simulink model "PV_Array_With_Faults"  (R2023b)
settings: Solver=FixedStepAuto  StartTime=1  StopTime=1440  FixedStep=1  RelTol=1e-3
libraries: spsSeriesRLCBranchLib x5, spsIdealSwitchLib x3, spsCurrentMeasurementLib x1, spsDiodeLib x1, spsMosfetLib x1, spsPVArrayLib x1, eePwmGenerator x1, spsVoltageMeasurementLib x1, spspowerguiLib x1
settings Model: NumberOfSteps=10  Creator=chate  LastModifiedBy=chate

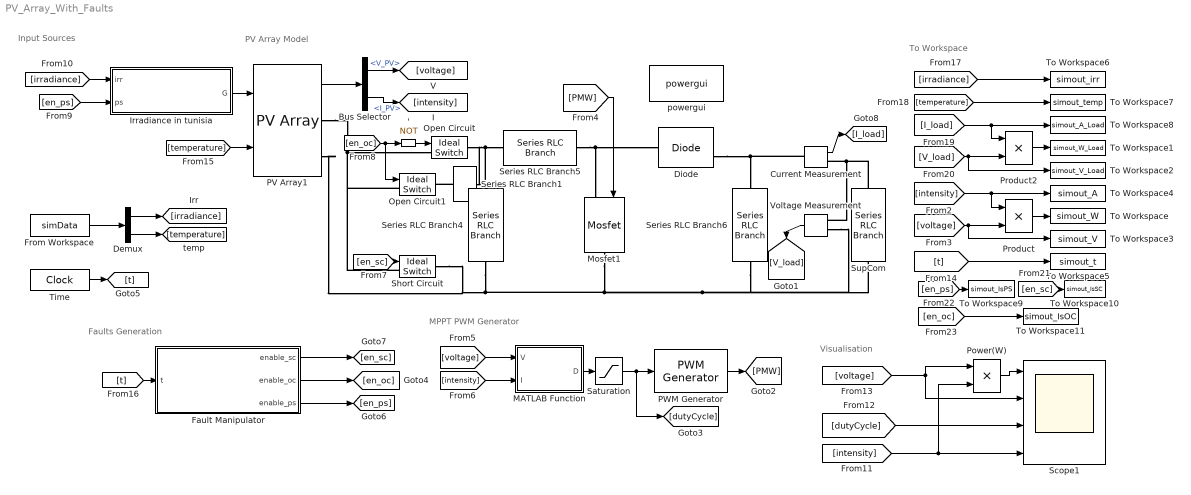
== system PV_Array_With_Faults ==
  note: Input Sources
  note: PV Array Model
  note: Faults Generation
  note: To Workspace
  note: MPPT PWM Generator
  note: Visualisation
  ' : Logic  Operator=NOT  IconShape=distinctive  AllPortsSameDT=off  OutDataTypeStr=boolean
  Bus Selector : BusSelector  OutputSignals=V_PV,I_PV
  Current Measurement : spsCurrentMeasurementLib/Current Measurement  PhasorSimulation=off  OutputType=Complex  PSBequivalent=0
  Demux : Demux  Outputs=2
  Diode : spsDiodeLib/Diode  Ron=0.001  Lon=0  Vf=0.8  IC=0  UseSnubber=0  Rs=100  Cs=1e-7  Measurements=on
  Fault Manipulator : MATLAB Function  TreatAsAtomicUnit=on
  From Workspace : FromWorkspace  VariableName=simData  OutputAfterFinalValue=Setting to zero
  Irradiance in tunisia : MATLAB Function  TreatAsAtomicUnit=on
  MATLAB Function : MATLAB Function  TreatAsAtomicUnit=on
  Mosfet1 : spsMosfetLib/Mosfet  Ron=1e-3  Lon=0  Rd=1e-3  Vfd=0  IC=0  Rs=100  Cs=1e-7  Measurements=off
  Open Circuit : spsIdealSwitchLib/Ideal Switch  Ron=0.000001  Lon=0  IC=1  Rs=0  Cs=0  Measurements=off
  Open Circuit1 : spsIdealSwitchLib/Ideal Switch  Ron=0.000001  Lon=0  IC=0  Rs=0  Cs=0  Measurements=off
  PV Array1 : spsPVArrayLib/PV Array  Npar=3  Nser=15  PlotType=array @ 1000 W/m2 & specified temperatures  S_vec="[ 1000  500  100 ]"  Temp_C_vec="[ 45 25  ]"  ModuleName=User-defined  PlotWhenSelected=off  Pm=451.278  Ncell=60  Voc=49.8  Isc=11.56  Vm=41.1  Im=10.98  beta_Voc_pc=-0.36099  alpha_Isc_pc=0.102  beta_Voc=-0.17977  alpha_Isc=0.011791  IL=11.6189  I0=4.2897e-10  nI=1.3452  Rsh=602.3017  Rs=0.22981  RobustModel=off  RobustCellTemperature=25  BAL=on  Tc=1e-6  Tfilter=5e-5
  PWM Generator : eePwmGenerator/PWM Generator  CarrCount=Up  Tper=864000  Tdelay=0  Ts=86400
  Power(W) : Product
  Product : Product
  Product2 : Product
  Saturation : Saturate  UpperLimit=1  LowerLimit=0
  Scope1 : Scope  NumInputPorts=4
  Series RLC Branch1 : spsSeriesRLCBranchLib/Series RLC Branch  LConnTagsString=__new0  RConnTagsString=__new0  BranchType=R  Resistance=7.3  Inductance=1.63e-2  SetiL0=off  InitialCurrent=0  Capacitance=1e-3  Setx0=off  InitialVoltage=0  Measurements=None
  Series RLC Branch4 : spsSeriesRLCBranchLib/Series RLC Branch  LConnTagsString=__new0  RConnTagsString=__new0  BranchType=C  Resistance=1  Inductance=1e-3  SetiL0=off  InitialCurrent=0  Capacitance=46.6e-2  Setx0=off  InitialVoltage=0  Measurements=None
  Series RLC Branch5 : spsSeriesRLCBranchLib/Series RLC Branch  LConnTagsString=__new0  RConnTagsString=__new0  BranchType=L  Resistance=1  Inductance=1.63e-2  SetiL0=off  InitialCurrent=0  Capacitance=1e-3  Setx0=off  InitialVoltage=0  Measurements=None
  Series RLC Branch6 : spsSeriesRLCBranchLib/Series RLC Branch  LConnTagsString=__new0  RConnTagsString=__new0  BranchType=C  Resistance=1  Inductance=1e-3  SetiL0=off  InitialCurrent=0  Capacitance=63e-2  Setx0=off  InitialVoltage=0  Measurements=None
  Short Circuit : spsIdealSwitchLib/Ideal Switch  Ron=0.000001  Lon=0  IC=0  Rs=0  Cs=0  Measurements=off
  SupCom : spsSeriesRLCBranchLib/Series RLC Branch  LConnTagsString=__new0  RConnTagsString=__new0  BranchType=R  Resistance=18.5  Inductance=1e-3  SetiL0=off  InitialCurrent=0  Capacitance=1e-3  Setx0=off  InitialVoltage=0  Measurements=None
  Time : DigitalClock
  To Workspace : ToWorkspace  VariableName=simout_W  SaveFormat=Timeseries  SampleTime=-1
  To Workspace1 : ToWorkspace  VariableName=simout_W_Load  SaveFormat=Timeseries  SampleTime=-1
  To Workspace10 : ToWorkspace  VariableName=simout_IsSC  SaveFormat=Timeseries  SampleTime=-1
  To Workspace11 : ToWorkspace  VariableName=simout_IsOC  SaveFormat=Timeseries  SampleTime=-1
  To Workspace2 : ToWorkspace  VariableName=simout_V_Load  SaveFormat=Timeseries  SampleTime=-1
  To Workspace3 : ToWorkspace  VariableName=simout_V  SaveFormat=Timeseries  SampleTime=-1
  To Workspace4 : ToWorkspace  VariableName=simout_A  SaveFormat=Timeseries  SampleTime=-1
  To Workspace5 : ToWorkspace  VariableName=simout_t  SaveFormat=Timeseries  SampleTime=-1
  To Workspace6 : ToWorkspace  VariableName=simout_irr  SaveFormat=Timeseries  SampleTime=-1
  To Workspace7 : ToWorkspace  VariableName=simout_temp  SaveFormat=Timeseries  SampleTime=-1
  To Workspace8 : ToWorkspace  VariableName=simout_A_Load  SaveFormat=Timeseries  SampleTime=-1
  To Workspace9 : ToWorkspace  VariableName=simout_IsPS  SaveFormat=Timeseries  SampleTime=-1
  Voltage Measurement : spsVoltageMeasurementLib/Voltage Measurement  PhasorSimulation=off  OutputType=Complex  PSBequivalent=0
  powergui : spspowerguiLib/powergui  Priority=1  SimulationMode=Discrete  SampleTime=1  frequency=60  Iterations=50  frequencyindice=0  Pbase=100e6  ErrMax=1e-4  UnitsV=kV  UnitsW=MW  buscounter=0  FunctionMessages=off  echomessages=off  EnableUseOfTLC=off  CurrentSourceSwitches=off  DisableSnubberDevices=off  DisableRonSwitches=off  DisableVfSwitches=off  DisplayEquations=off  AutomaticDiscreteSolvers=off  SolverType=Tustin/Backward Euler (TBE)  Interpol=off  ExternalGateDelay=off  methode=off  Ts=100  x0status=blocks  SPID=on  SwTol=0  HookPort=off  NonlinearTolerance=1e-4  nMaxIteration=100  ContinueOnMaxIteration=off  RestoreLinks=warning  ResistiveCurrentMeasurement=off  Frange=[0:2:500]  Ylog=off  Xlog=on  ShowGrid=off  save=off  variable=ZData  structure=0  ZoomFFT=off  StartTime=0.0  cycles=1  DisplayStyle=1  fundamental=60  FreqAxis=off  MaxFrequency=1000  frequencyindicesteady=1  RmsSteady=1  display=off
  wires:
  PV Array1/1 -> Bus Selector/1
  [intensity] -> Product/1, To Workspace4/1
  [voltage] -> To Workspace3/1, Product/2
  Product/1 -> To Workspace/1
  Bus Selector/1 -> [voltage]  "<V_PV>"
  Bus Selector/2 -> [intensity]  "<I_PV>"
  Voltage Measurement/1 -> [V_load]
  [PMW] -> Mosfet1/1
  MATLAB Function/1(D) -> Saturation/1
  PWM Generator/1 -> [PMW]
  [voltage] -> MATLAB Function/1(V)
  [intensity] -> MATLAB Function/2(I)
  [dutyCycle] -> Scope1/3
  [voltage] -> Power(W)/1, Scope1/2
  Power(W)/1 -> Scope1/1
  [intensity] -> Power(W)/2, Scope1/4
  Saturation/1 -> PWM Generator/1, [dutyCycle]
  Irradiance in tunisia/1(G) -> PV Array1/1
  [en_sc] -> Short Circuit/1
  Fault Manipulator/2(enable_oc) -> [en_oc]
  Fault Manipulator/1(enable_sc) -> [en_sc]
  [en_ps] -> Irradiance in tunisia/2(ps)
  Fault Manipulator/3(enable_ps) -> [en_ps]
  Time/1 -> [t]
  [t] -> To Workspace5/1
  [t] -> Fault Manipulator/1(t)
  Current Measurement/1 -> [I_load]
  [irradiance] -> To Workspace6/1
  [temperature] -> To Workspace7/1
  [V_load] -> To Workspace2/1, Product2/2
  Product2/1 -> To Workspace1/1
  [I_load] -> Product2/1, To Workspace8/1
  [en_ps] -> To Workspace9/1
  [en_sc] -> To Workspace10/1
  [en_oc] -> To Workspace11/1
  From Workspace/1 -> Demux/1
  Demux/2 -> [temperature]
  [temperature] -> PV Array1/2
  Demux/1 -> [irradiance]
  [irradiance] -> Irradiance in tunisia/1(irr)
  [en_oc] -> '/1, Open Circuit1/1
  '/1 -> Open Circuit/1
  connections:
  SupCom/LConn1 -- Current Measurement/RConn1 -- Voltage Measurement/LConn1
  Series RLC Branch4/RConn1 -- Short Circuit/RConn1 -- PV Array1/RConn2 -- Series RLC Branch6/RConn1 -- Voltage Measurement/LConn2 -- SupCom/RConn1 -- Mosfet1/RConn1
  Series RLC Branch5/RConn1 -- Mosfet1/LConn1 -- Diode/LConn1
  Current Measurement/LConn1 -- Diode/RConn1 -- Series RLC Branch6/LConn1
  Series RLC Branch4/LConn1 -- Series RLC Branch1/RConn1 -- Open Circuit/RConn1 -- Series RLC Branch5/LConn1
  PV Array1/RConn1 -- Open Circuit1/LConn1 -- Short Circuit/LConn1 -- Open Circuit/LConn1
  Series RLC Branch1/LConn1 -- Open Circuit1/RConn1

== matlab function PV_Array_With_Faults/Irradiance in tunisia ==
  data: irr input; G output; ps input
function G = irradiance_in_tunisia(irr, ps)
    
    G = max(0, irr);

    if ps == 1
        G = 0.85 * G;  % Reduce irradiance to 85%
    end
end

== matlab function PV_Array_With_Faults/Fault Manipulator ==
  data: t input; enable_sc output; enable_oc output; enable_ps output
function [enable_sc, enable_oc, enable_ps] = faults(t)
    % Time-dependent fault trigger system
    % Fault probability per second
    persistent fault_type fault_start_time fault_duration

    % Parameters
    fault_probability = 0.05;  % chance of a fault occurring at each call
    enable_sc = 0;
    enable_oc = 0;
    enable_ps = 0;

    % First call init
    if isempty(fault_type)
        fault_type = 0;
        fault_duration = 0;
        fault_start_time = -Inf;
    end

    % Check if current fault is active
    if t < fault_start_time + fault_duration
        % Maintain the current fault
        switch fault_type
            case 1
                enable_sc = 1;
                enable_oc = 0;
                enable_ps = 0;
            case 2
                enable_sc = 0;
                enable_oc = 1;
                enable_ps = 0;
            case 3
                enable_sc = 0;
                enable_oc = 0;
                enable_ps = 1;
        end
    else
        % No active fault, decide if a new one should start
        if rand < fault_probability
            fault_duration = randi(50) + 10;
            fault_type = randi(3);  % random fault (1=SC, 2=OC, 3=PS)
            fault_start_time = t;
        else
            % No fault
            fault_type = 0;
            enable_sc = 0;
            enable_oc = 0;
            enable_ps = 0;
        end
    end
end

== matlab function PV_Array_With_Faults/MATLAB Function ==
  data: V input; D output; I input
function D = MPPT(V, I)
    persistent Vold Pold Dold;

    % MPPT parameters
    deltaD = 0.005;    % Step size
    P = V * I;
    
    % Initialize with better startup conditions
    if isempty(Vold)
        Vold = V;
        Pold = P;
        Dold = 0.175;  % Starting duty cycle
    end
    
    % Startup protection
    if V < 10  % If voltage is too low
        D = 0.05;  % Minimum duty cycle to build up voltage
        
        % Update persistent variables
        Vold = V;
        Pold = P;
        Dold = D;
        return;
    end
    
    % Modified P&O algorithm with additional checks
    if abs(V - Vold) < 0.1  % If voltage barely changed
        deltaD = 0.01;  % Increase step size
    end

    if (P - Pold) ~= 0
        if (P - Pold) > 0
            if (V - Vold) > 0
                D = Dold + deltaD;
            else
                D = Dold - deltaD;
            end
        else
            if (V - Vold) > 0
                D = Dold - deltaD;
            else
                D = Dold + deltaD;
            end
        end
    else
        D = Dold;
    end
    
    % Update old values
    Vold = V;
    Pold = P;
    Dold = D;
    D = max(min(D, 2000), 0.05);
end
